simulink model "unitstepdisturbance"  (R2021b)
settings: Solver=VariableStepAuto  StartTime=0.0  StopTime=100  RelTol=1e-3
settings Model: Creator=Asus  LastModifiedBy=Matina Kaviani
settings SolverCC: AlgebraicLoopSolver=TrustRegion
settings DebuggingCC: SFMachineParentedDataDiag=warning

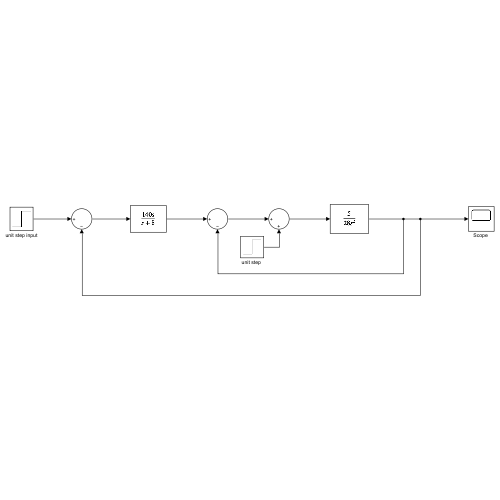
[thumbnail: Simulink's stored preview of the top-level diagram]
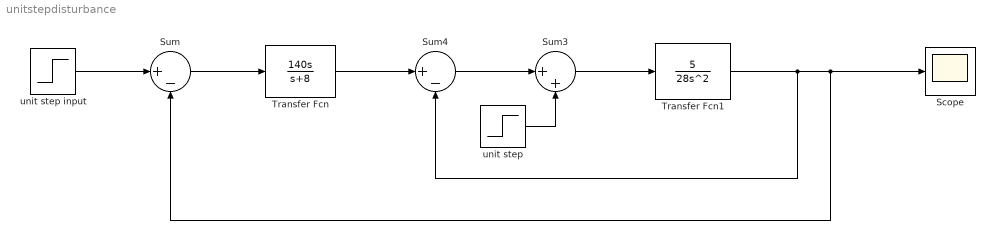
== system unitstepdisturbance ==
  "Scope " : Scope
  Sum : Sum  Inputs=|+-
  Sum3 : Sum  Inputs=|++
  Sum4 : Sum  Inputs=|+-
  Transfer Fcn : TransferFcn  Numerator=[140 0]  Denominator=[1 8]
  Transfer Fcn1 : TransferFcn  Numerator=[0 5]  Denominator=[28 0 0]
  "unit step " : Step  SampleTime=0
  unit step input : Step  SampleTime=0
  wires:
  unit step input/1 -> Sum/1
  Sum/1 -> Transfer Fcn/1
  Transfer Fcn/1 -> Sum4/1
  Sum4/1 -> Sum3/1
  Sum3/1 -> Transfer Fcn1/1
  "unit step "/1 -> Sum3/2
  Transfer Fcn1/1 -> Sum4/2, Sum/2, "Scope "/1
